simulink model "MPU6050"  (R2019b)
settings: Solver=FixedStepDiscrete  StartTime=0.0  StopTime=inf  FixedStep=0.05  RelTol=1e-3  EnableMultiTasking=on
InitFcn:
  | Ts=0.05;
  | AccScale=4;
  | GyroScale=1000;
libraries: arduinolib x2
settings Model: SimulationMode=external  SILPILModeSetting=veronly  ExtModeTrigDuration=2  Creator=Marc  LastModifiedBy=vuwij
settings DataIOCC: SaveOutput=off  SaveTime=off  ReturnWorkspaceOutputs=off  TimeSaveName=time
settings OptimizationCC: LifeSpan=1  MaxStackSize=64
settings DebuggingCC: AllowSymbolicDim=off  SFUnexpectedBacktrackingDiag=warning  SFNoUnconditionalDefaultTransitionDiag=warning  ArithmeticOperatorsInVariantConditions=warning
settings HardwareCC: ProdBitPerInt=16  ProdBitPerPointer=16  ProdBitPerSizeT=16  ProdBitPerPtrDiffT=16  ProdLargestAtomicFloat=None  ProdWordSize=8  ProdHWDeviceType=Atmel->AVR
settings ModelReferenceCC: PropagateSignalLabelsOutOfModel=off
settings SFSimCC: SimUseLocalCustomCode=off  CustomCodeUndefinedFunction=UseInterfaceOnly
settings RTWCC: SystemTargetFile=ert.tlc  HardwareBoard=Arduino Nano 3.0  TemplateMakefile=ert_default_tmf  RTWUseLocalCustomCode=off  Toolchain=Arduino AVR  BuildConfiguration=Faster Runs
settings CodeAppCC: MangleLength=10  StateflowObjectComments=on
settings ERTTargetCC: MultiwordLength=2048  ERTCustomFileBanners=off  SupportContinuousTime=on  SupportNonInlinedSFcns=on  SupportVariableSizeSignals=on  ModelStepFunctionPrototypeControlCompliant=off  ExtModeStaticAllocSize=250  ConvertIfToSwitch=off  SuppressUnreachableDefaultCases=off
settings ConfigComp: CovMetricSettings=dw  CovHtmlReporting=on  CovSaveCumulativeToWorkspaceVar=on  CovSaveSingleToWorkspaceVar=on  CovExternalEMLEnable=off
settings SimscapeCC: SimscapeNormalizeSystem=off

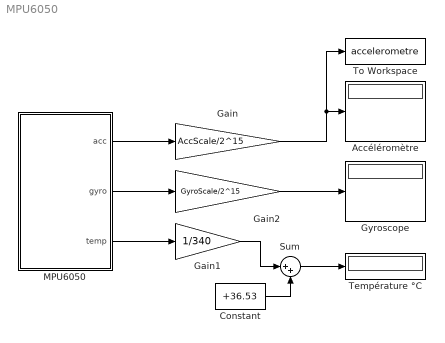
== system MPU6050 ==
  Accéléromètre : Display
  Constant : Constant  Value=+36.53  OutDataTypeStr=single
  Gain : Gain  Gain=AccScale/2^15  OutDataTypeStr=single
  Gain1 : Gain  Gain=1/340  OutDataTypeStr=single
  Gain2 : Gain  Gain=GyroScale/2^15  OutDataTypeStr=single
  Gyroscope : Display
  MPU6050 : Stateflow chart  TreatAsAtomicUnit=on
  Sum : Sum  Inputs=|++
  Température °C : Display
  To Workspace : ToWorkspace  VariableName=accelerometre  SampleTime=Ts
  wires:
  Gain/1 -> Accéléromètre/1, To Workspace/1
  MPU6050/1(acc) -> Gain/1
  MPU6050/2(gyro) -> Gain2/1
  Gain2/1 -> Gyroscope/1
  MPU6050/3(temp) -> Gain1/1
  Gain1/1 -> Sum/1
  Constant/1 -> Sum/2
  Sum/1 -> Température °C/1

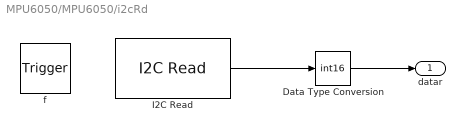
== system MPU6050/MPU6050/i2cRd ==
  f : TriggerPort  TriggerType=function-call  VariantControl=Variant  SampleTimeType=periodic  SampleTime=-1
      settings: CopyFcn=Stateflow.SLINSF.SimulinkMan.removeBlockPreDeleteFcn  PreDeleteFcn=Stateflow.SLINSF.SimulinkMan.unsafePredeleteFcn
  Data Type Conversion : DataTypeConversion  OutDataTypeStr=int16
  I2C Read : arduinolib/I2C Read  I2CModule=0  Mode=Master  SlaveAddress=hex2dec( '68' )  SlaveByteOrder=BigEndian  Direction=Receiver  RegisterAddressMode=on  RegisterAddress=hex2dec( '3b' )  SlaveDataType=uint16  DataLength=7  NoAck=off  RepeatedStart=off  OutputStatus=off  blockPlatform=arduino  SampleTime=-1
      settings: SourceProductName=Simulink Support Package for Arduino Hardware  SourceProductBaseCode=ARDUINO
  datar : Outport  OutDataTypeStr=int16  Unit=1  PortDimensions=7  SampleTime=Ts
  wires:
  I2C Read/1 -> Data Type Conversion/1
  Data Type Conversion/1 -> datar/1

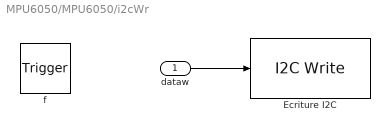
== system MPU6050/MPU6050/i2cWr ==
  dataw : Inport  OutDataTypeStr=uint16  Unit=1  PortDimensions=1
  f : TriggerPort  TriggerType=function-call  VariantControl=Variant  SampleTimeType=periodic  SampleTime=-1
      settings: CopyFcn=Stateflow.SLINSF.SimulinkMan.removeBlockPreDeleteFcn  PreDeleteFcn=Stateflow.SLINSF.SimulinkMan.unsafePredeleteFcn
  Ecriture I2C : arduinolib/I2C Write  Priority=1  I2CModule=0  Mode=Master  SlaveAddress=hex2dec( '68' )  SlaveByteOrder=BigEndian  Direction=Transmitter  RegisterAddressMode=off  RegisterAddress=hex2dec( '6B' )  SlaveDataType=uint16  DataLength=1  NoAck=off  RepeatedStart=off  OutputStatus=off  blockPlatform=arduino
      settings: SourceProductName=Simulink Support Package for Arduino Hardware  SourceProductBaseCode=ARDUINO
  wires:
  dataw/1 -> Ecriture I2C/1

== stateflow chart MPU6050/MPU6050 ==
  state initialisation
    en:
    i2cWr(uint16(hex2dec( '6B00' )));%Power on
    i2cWr(uint16(hex2dec( '1B10' )));%gyro 0x10=1000°/s
    i2cWr(uint16(hex2dec( '1C08' )));%acce 0x08= 4G
    i2cWr(uint16(hex2dec( '1A06' )));%filtrage+actu 0x06= 19ms
    i2cWr(uint16(hex2dec( '3710' )));%INT_PIN_CFG
    i2cWr(uint16(hex2dec( '3800' )));%Interrupt Enable 0 désactivé
  state i2cWr(dataw) [function]
  state datar = i2cRd [function]
  state Lecture_acceleration3_axes
    during:
    val=i2cRd;
    acc=val(1:3);
    gyro=val(5:7);
    temp=val(4:4);
  (default) -> initialisation
  initialisation -> Lecture_acceleration3_axes
  data: dataw function_input uint16 size=1; datar function_output int16 size=7; acc output int16 size=3; n local uint8 size=1; gyro output int16 size=3; val local int16 size=7; temp output int16 size=1
